simulink library "aerolibtransform"  (Simulink 5.0)
libraries: simulink x5, aerolibtransform x2, aerolibutil x2, simulink3 x1
settings Model: Creator=sgage  LastModifiedBy=sgage  ExtModeAutoUpdateStatusClock=off  TargetHWChar=2  TargetHWWordLengths=8,16,32,32
settings Model: ForwardingTableString=|
  | ||__slOldName__||aerolibtransform/Direction Cosine Matrix to
  | Euler Angles||__slNewName__||aerolibtransform2/Direction Cosine Matrix to
  | Euler Angles||__slOldName__||aerolibtransform/Euler Angles to
  | Direction Cosine Matrix||__slNewName__||aerolibtransform2/Euler Angles to
  | Direction Cosine Matrix||__slOldName__||aerolibtransform/Direction Cosine Matrix
  | to Quaternions||__slNewName__||aerolibtransform2/Direction Cosine Matrix
  | to Quaternions||__slOldName__||aerolibtransform/Quaternions to
  | Direction Cosine Matrix||__slNewName__||aerolibtransform2/Quaternions to
  | Direction Cosine Matrix||__slOldName__||aerolibtransform/Euler Angles to Quaternions||__slNewName__||aerolibtransform2/Euler Angles to Quaternions||__slOldName__||aerolibtransform/Quaternions to Euler Angles||__slNewName__||aerolibtransform2/Quaternions to Euler Angles||__slOldName__||aerolibtransform/3x3 Cross Product||__slNewName__||aerolibutil/3x3 Cross Product

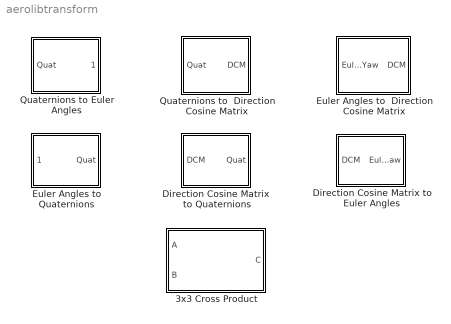
== system aerolibtransform ==
  3x3 Cross Product : Subsystem
      mask Type: CrossProduct
      mask Description: Calculate the cross product of two 3-by-1 vectors.
      mask Help: web(asbhelp('3x3crossproduct'));
      mask Display: disp('Cross Product \n C = AxB')
  Direction Cosine Matrix  to Quaternions : Subsystem
      mask Type: DCM2Quaternion
      mask Description: Determine the 4x1 quaternion orientation vector from a 3-by-3 direction cosine matrix (DCM). The input DCM transforms vectors from inertial axes to body axes.
      mask Help: web(asbhelp('directioncosinematrixtoquaternions'));
      mask Display: disp('DCM2Quat')
  Direction Cosine Matrix to Euler Angles : Subsystem
      mask Type: DCM2Euler
      mask Description: Determine an euler orientation (roll, pitch, yaw) from the 3-by-3 direction cosine matrix (DCM). The input DCM transforms vectors from inertial axes to body axes.
      mask Help: web(asbhelp('directioncosinematrixtoeulerangles'));
      mask Display: disp('DCM2Eul')
  Euler Angles to  Direction Cosine Matrix : Subsystem
      mask Type: Euler2DCM
      mask Description: Determine the 3-by-3 direction cosine matrix (DCM) from an Euler orientation (roll, pitch, yaw). The output DCM transforms vectors from inertial axes to body axes.
      mask Help: web(asbhelp('euleranglestodirectioncosinematrix'));
      mask Display: disp('Eul2DCM')
  Euler Angles to Quaternions : Subsystem
      mask Type: Euler2Quaternion
      mask Description: Calculate quaternion (q0,q1,q2,q3) from Euler angles (roll, pitch, yaw)
      mask Help: web(asbhelp('euleranglestoquaternions'));
      mask Display: disp('Eul2Quat')
  Quaternions to  Direction Cosine Matrix : Subsystem
      mask Type: Quaternion2DCM
      mask Description: Determine the 3-by-3 direction cosine matrix (DCM) from a 4-by-1 quaternion orientation vector. The output DCM transforms vectors from inertial axes to body axes.
      mask Help: web(asbhelp('quaternionstodirectioncosinematrix'));
      mask Display: disp('Quat2DCM')
  Quaternions to Euler Angles : Subsystem
      mask Type: Quaternion2Euler
      mask Description: Calculate Euler angles (roll, pitch, yaw) from quaternion (q0,q1,q2,q3)
      mask Help: web(asbhelp('quaternionstoeulerangles'));
      mask Display: disp('Quat2Eul')

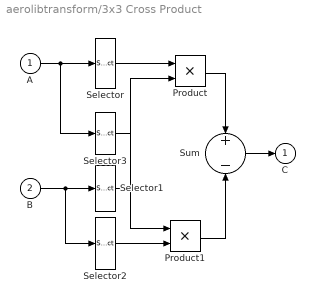
== system aerolibtransform/3x3 Cross Product ==
  A : Inport
  B : Inport  Port=2
  Product : Product  SaturateOnIntegerOverflow=on  InputSameDT=on
  Product1 : Product  SaturateOnIntegerOverflow=on  InputSameDT=on
  Selector : Selector  Elements=[2 3 1]  InputPortWidth=3
  Selector1 : Selector  Elements=[3 1 2]  InputPortWidth=3
  Selector2 : Selector  Elements=[2 3 1]  InputPortWidth=3
  Selector3 : Selector  Elements=[3 1 2]  InputPortWidth=3
  Sum : Sum  Inputs=+|-  SaturateOnIntegerOverflow=on  InputSameDT=on
  C : Outport  InitialOutput=0
  wires:
  Selector3/1 -> Product1/1
  Selector2/1 -> Product1/2
  Product1/1 -> Sum/2
  Selector1/1 -> Product/2
  Product/1 -> Sum/1
  A/1 -> Selector3/1, Selector/1
  Selector/1 -> Product/1
  B/1 -> Selector2/1, Selector1/1
  Sum/1 -> C/1

== system aerolibtransform/Direction Cosine Matrix  to Quaternions ==
  DCM : Inport
  If : If
  Merge : Merge
  Negative Trace : Subsystem  TreatAsAtomicUnit=on
  Positive Trace : Subsystem  TreatAsAtomicUnit=on
  "Reshape 3x3 -> 9x1" : simulink/Math Operations/Reshape  OutputDimensionality=Customize  OutputDimensions=[9,1]
  trace(DCM) : Fcn  Expr=u(1)+u(5)+u(9)
  Quat : Outport
  wires:
  If/2 -> Negative Trace/Action
  If/1 -> Positive Trace/Action
  Negative Trace/1(qw qx qy qz) -> Merge/2
  DCM/1 -> "Reshape 3x3 -> 9x1"/1
  "Reshape 3x3 -> 9x1"/1 -> trace(DCM)/1, Positive Trace/2(DCM), Negative Trace/1(DCM)
  trace(DCM)/1 -> If/1, Positive Trace/1(trace(DCM))
  Positive Trace/1(qw qx qy qz) -> Merge/1
  Merge/1 -> Quat/1

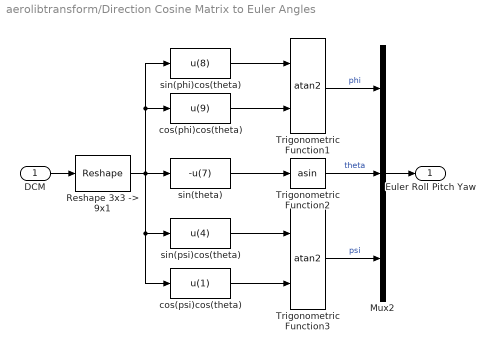
== system aerolibtransform/Direction Cosine Matrix to Euler Angles ==
  DCM : Inport
  Mux2 : Mux  Inputs=3
  "Reshape 3x3 -> 9x1" : simulink/Math Operations/Reshape  OutputDimensionality=Customize  OutputDimensions=[9, 1]
  Trigonometric Function1 : Trigonometry  Operator=atan2
  Trigonometric Function2 : Trigonometry  Operator=asin
  Trigonometric Function3 : Trigonometry  Operator=atan2
  cos(phi)cos(theta) : Fcn  Expr=u(9)
  cos(psi)cos(theta) : Fcn  Expr=u(1)
  sin(phi)cos(theta) : Fcn  Expr=u(8)
  sin(psi)cos(theta) : Fcn  Expr=u(4)
  sin(theta) : Fcn  Expr=-u(7)
  Euler Roll Pitch Yaw : Outport  InitialOutput=0
  wires:
  Mux2/1 -> Euler Roll Pitch Yaw/1
  Trigonometric Function3/1 -> Mux2/3  "psi"
  Trigonometric Function2/1 -> Mux2/2  "theta"
  Trigonometric Function1/1 -> Mux2/1  "phi"
  cos(psi)cos(theta)/1 -> Trigonometric Function3/2
  sin(psi)cos(theta)/1 -> Trigonometric Function3/1
  cos(phi)cos(theta)/1 -> Trigonometric Function1/2
  sin(phi)cos(theta)/1 -> Trigonometric Function1/1
  sin(theta)/1 -> Trigonometric Function2/1
  "Reshape 3x3 -> 9x1"/1 -> cos(psi)cos(theta)/1, sin(psi)cos(theta)/1, cos(phi)cos(theta)/1, sin(phi)cos(theta)/1, sin(theta)/1
  DCM/1 -> "Reshape 3x3 -> 9x1"/1

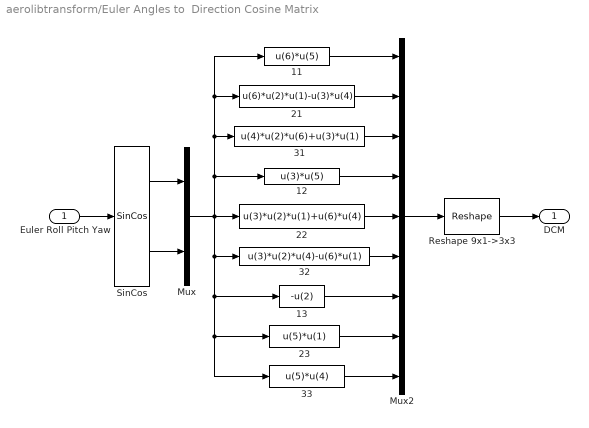
== system aerolibtransform/Euler Angles to  Direction Cosine Matrix ==
  Euler Roll Pitch Yaw : Inport
  11 : Fcn  Expr=u(6)*u(5)
  12 : Fcn  Expr=u(3)*u(5)
  13 : Fcn  Expr=-u(2)
  21 : Fcn  Expr=u(6)*u(2)*u(1)-u(3)*u(4)
  22 : Fcn  Expr=u(3)*u(2)*u(1)+u(6)*u(4)
  23 : Fcn  Expr=u(5)*u(1)
  31 : Fcn  Expr=u(4)*u(2)*u(6)+u(3)*u(1)
  32 : Fcn  Expr=u(3)*u(2)*u(4)-u(6)*u(1)
  33 : Fcn  Expr=u(5)*u(4)
  Mux : Mux  Inputs=2
  Mux2 : Mux  Inputs=9
  Reshape 9x1->3x3 : simulink/Math Operations/Reshape  OutputDimensionality=Customize  OutputDimensions=[3,3]
  SinCos : aerolibutil/SinCos
  DCM : Outport  InitialOutput=0
  wires:
  Mux/1 -> 33/1, 23/1, 13/1, 32/1, 12/1, 31/1, 21/1, 11/1, 22/1
  SinCos/2 -> Mux/2
  SinCos/1 -> Mux/1
  Reshape 9x1->3x3/1 -> DCM/1
  Mux2/1 -> Reshape 9x1->3x3/1
  11/1 -> Mux2/1
  21/1 -> Mux2/2
  31/1 -> Mux2/3
  12/1 -> Mux2/4
  22/1 -> Mux2/5
  32/1 -> Mux2/6
  13/1 -> Mux2/7
  23/1 -> Mux2/8
  33/1 -> Mux2/9
  Euler Roll Pitch Yaw/1 -> SinCos/1

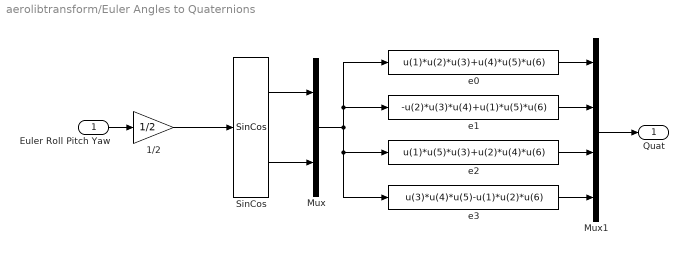
== system aerolibtransform/Euler Angles to Quaternions ==
  Euler Roll Pitch Yaw : Inport
  1/2 : Gain  Gain=1/2  SaturateOnIntegerOverflow=on
  Mux : Mux  Inputs=2
  Mux1 : Mux
  SinCos : aerolibutil/SinCos
  e0 : Fcn  Expr=u(1)*u(2)*u(3)+u(4)*u(5)*u(6)
  e1 : Fcn  Expr=-u(2)*u(3)*u(4)+u(1)*u(5)*u(6)
  e2 : Fcn  Expr=u(1)*u(5)*u(3)+u(2)*u(4)*u(6)
  e3 : Fcn  Expr=u(3)*u(4)*u(5)-u(1)*u(2)*u(6)
  Quat : Outport  InitialOutput=0
  wires:
  Mux1/1 -> Quat/1
  e3/1 -> Mux1/4
  e2/1 -> Mux1/3
  e1/1 -> Mux1/2
  e0/1 -> Mux1/1
  Mux/1 -> e0/1, e1/1, e3/1, e2/1
  SinCos/2 -> Mux/2
  SinCos/1 -> Mux/1
  Euler Roll Pitch Yaw/1 -> 1/2/1
  1/2/1 -> SinCos/1

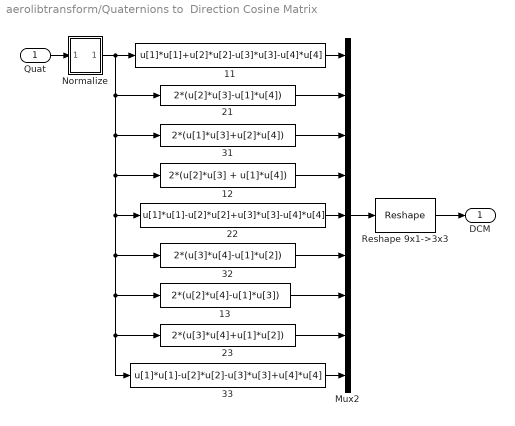
== system aerolibtransform/Quaternions to  Direction Cosine Matrix ==
  Quat : Inport
  11 : Fcn  Expr=u[1]*u[1]+u[2]*u[2]-u[3]*u[3]-u[4]*u[4]
  12 : Fcn  Expr=2*(u[2]*u[3] + u[1]*u[4])
  13 : Fcn  Expr=2*(u[2]*u[4]-u[1]*u[3])
  21 : Fcn  Expr=2*(u[2]*u[3]-u[1]*u[4])
  22 : Fcn  Expr=u[1]*u[1]-u[2]*u[2]+u[3]*u[3]-u[4]*u[4]
  23 : Fcn  Expr=2*(u[3]*u[4]+u[1]*u[2])
  31 : Fcn  Expr=2*(u[1]*u[3]+u[2]*u[4])
  32 : Fcn  Expr=2*(u[3]*u[4]-u[1]*u[2])
  33 : Fcn  Expr=u[1]*u[1]-u[2]*u[2]-u[3]*u[3]+u[4]*u[4]
  Mux2 : Mux  Inputs=9
  Normalize : Subsystem
  Reshape 9x1->3x3 : simulink/Math Operations/Reshape  OutputDimensionality=Customize  OutputDimensions=[3,3]
  DCM : Outport  InitialOutput=0
  wires:
  Mux2/1 -> Reshape 9x1->3x3/1
  Reshape 9x1->3x3/1 -> DCM/1
  11/1 -> Mux2/1
  21/1 -> Mux2/2
  31/1 -> Mux2/3
  12/1 -> Mux2/4
  22/1 -> Mux2/5
  32/1 -> Mux2/6
  13/1 -> Mux2/7
  23/1 -> Mux2/8
  33/1 -> Mux2/9
  Quat/1 -> Normalize/1(In1)
  Normalize/1(Out1) -> 11/1, 21/1, 31/1, 12/1, 22/1, 32/1, 13/1, 33/1, 23/1

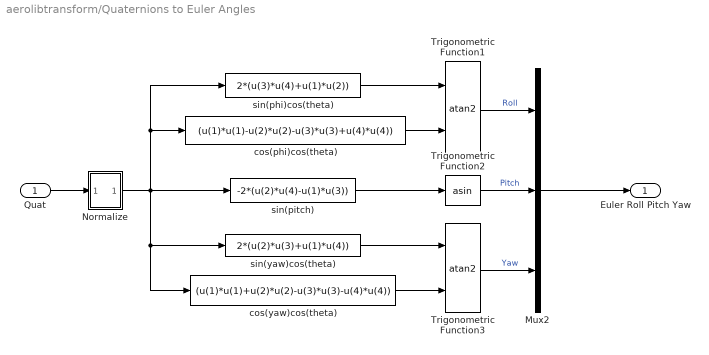
== system aerolibtransform/Quaternions to Euler Angles ==
  Quat : Inport
  Mux2 : Mux  Inputs=3
  Normalize : Subsystem
  Trigonometric Function1 : Trigonometry  Operator=atan2
  Trigonometric Function2 : Trigonometry  Operator=asin
  Trigonometric Function3 : Trigonometry  Operator=atan2
  cos(phi)cos(theta) : Fcn  Expr=(u(1)*u(1)-u(2)*u(2)-u(3)*u(3)+u(4)*u(4))
  cos(yaw)cos(theta) : Fcn  Expr=(u(1)*u(1)+u(2)*u(2)-u(3)*u(3)-u(4)*u(4))
  sin(phi)cos(theta) : Fcn  Expr=2*(u(3)*u(4)+u(1)*u(2))
  sin(pitch) : Fcn  Expr=-2*(u(2)*u(4)-u(1)*u(3))
  sin(yaw)cos(theta) : Fcn  Expr=2*(u(2)*u(3)+u(1)*u(4))
  Euler Roll Pitch Yaw : Outport  InitialOutput=0
  wires:
  Quat/1 -> Normalize/1(In1)
  Normalize/1(Out1) -> cos(phi)cos(theta)/1, sin(phi)cos(theta)/1, sin(pitch)/1, cos(yaw)cos(theta)/1, sin(yaw)cos(theta)/1
  Trigonometric Function2/1 -> Mux2/2  "Pitch"
  Mux2/1 -> Euler Roll Pitch Yaw/1
  sin(pitch)/1 -> Trigonometric Function2/1
  Trigonometric Function1/1 -> Mux2/1  "Roll"
  sin(phi)cos(theta)/1 -> Trigonometric Function1/1
  cos(phi)cos(theta)/1 -> Trigonometric Function1/2
  Trigonometric Function3/1 -> Mux2/3  "Yaw"
  sin(yaw)cos(theta)/1 -> Trigonometric Function3/1
  cos(yaw)cos(theta)/1 -> Trigonometric Function3/2

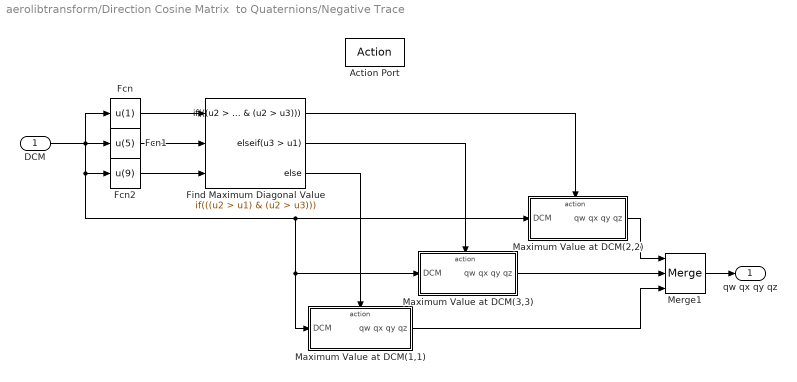
== system aerolibtransform/Direction Cosine Matrix  to Quaternions/Negative Trace ==
  DCM : Inport
  Action Port : ActionPort
  Fcn : Fcn  Expr=u(1)
  Fcn1 : Fcn  Expr=u(5)
  Fcn2 : Fcn  Expr=u(9)
  Find Maximum Diagonal Value : If  NumInputs=3  IfExpression=((u2 > u1) & (u2 > u3))  ElseIfExpressions=u3 > u1
  Maximum Value at DCM(1,1) : Subsystem  TreatAsAtomicUnit=on
  Maximum Value at DCM(2,2) : Subsystem  TreatAsAtomicUnit=on
  Maximum Value at DCM(3,3) : Subsystem  TreatAsAtomicUnit=on
  Merge1 : Merge  Inputs=3
  qw qx qy qz : Outport
  wires:
  Fcn2/1 -> Find Maximum Diagonal Value/3
  Fcn1/1 -> Find Maximum Diagonal Value/2
  Fcn/1 -> Find Maximum Diagonal Value/1
  DCM/1 -> Fcn2/1, Maximum Value at DCM(2,2)/1(DCM), Maximum Value at DCM(3,3)/1(DCM), Maximum Value at DCM(1,1)/1(DCM), Fcn1/1, Fcn/1
  Find Maximum Diagonal Value/3 -> Maximum Value at DCM(1,1)/Action
  Maximum Value at DCM(2,2)/1(qw qx qy qz) -> Merge1/1
  Maximum Value at DCM(3,3)/1(qw qx qy qz) -> Merge1/2
  Maximum Value at DCM(1,1)/1(qw qx qy qz) -> Merge1/3
  Merge1/1 -> qw qx qy qz/1
  Find Maximum Diagonal Value/1 -> Maximum Value at DCM(2,2)/Action
  Find Maximum Diagonal Value/2 -> Maximum Value at DCM(3,3)/Action

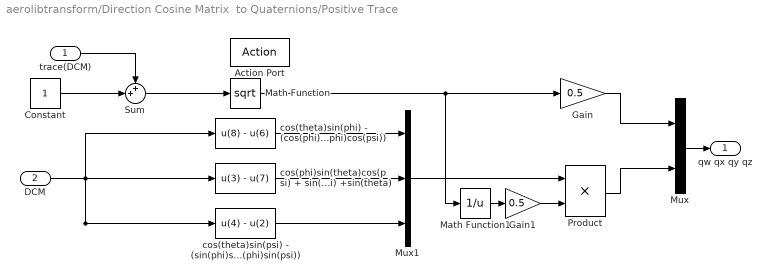
== system aerolibtransform/Direction Cosine Matrix  to Quaternions/Positive Trace ==
  trace(DCM) : Inport
  DCM : Inport  Port=2
  Action Port : ActionPort
  Constant : Constant  ShowAdditionalParam=on
  Gain : Gain  Gain=0.5  ShowAdditionalParam=on  SaturateOnIntegerOverflow=on
  Gain1 : Gain  Gain=0.5  ShowAdditionalParam=on  SaturateOnIntegerOverflow=on
  Math Function : Math  Operator=sqrt
  Math Function1 : Math  Operator=reciprocal
  Mux : Mux  Inputs=2
  Mux1 : Mux  Inputs=3
  Product : Product  ShowAdditionalParam=on  SaturateOnIntegerOverflow=on  InputSameDT=on
  Sum : Sum  Inputs=++|  ShowAdditionalParam=on  SaturateOnIntegerOverflow=on  InputSameDT=on
  cos(phi)sin(theta)cos(psi) + sin(phi)sin(psi) +sin(theta) : Fcn  Expr=u(3) - u(7)
  cos(theta)sin(phi) - (cos(phi)sin(theta)sin(psi) - sin(phi)cos(psi)) : Fcn  Expr=u(8) - u(6)
  cos(theta)sin(psi) - (sin(phi)sin(theta)cos(psi) - cos(phi)sin(psi)) : Fcn  Expr=u(4) - u(2)
  qw qx qy qz : Outport
  wires:
  Math Function/1 -> Gain/1, Math Function1/1
  Sum/1 -> Math Function/1
  Mux/1 -> qw qx qy qz/1
  cos(theta)sin(psi) - (sin(phi)sin(theta)cos(psi) - cos(phi)sin(psi))/1 -> Mux1/3
  cos(phi)sin(theta)cos(psi) + sin(phi)sin(psi) +sin(theta)/1 -> Mux1/2
  cos(theta)sin(phi) - (cos(phi)sin(theta)sin(psi) - sin(phi)cos(psi))/1 -> Mux1/1
  DCM/1 -> cos(theta)sin(phi) - (cos(phi)sin(theta)sin(psi) - sin(phi)cos(psi))/1, cos(phi)sin(theta)cos(psi) + sin(phi)sin(psi) +sin(theta)/1, cos(theta)sin(psi) - (sin(phi)sin(theta)cos(psi) - cos(phi)sin(psi))/1
  Math Function1/1 -> Gain1/1
  Gain/1 -> Mux/1
  Mux1/1 -> Product/1
  Gain1/1 -> Product/2
  Constant/1 -> Sum/2
  trace(DCM)/1 -> Sum/1
  Product/1 -> Mux/2

== system aerolibtransform/Quaternions to  Direction Cosine Matrix/Normalize ==
  In1 : Inport
  Dot Product : simulink/Math Operations/Dot Product
  Math Function : Math  Operator=sqrt
  Normalize Quaternion Magnitude : Product  Inputs=*/  SaturateOnIntegerOverflow=on  InputSameDT=on
  Out1 : Outport
  wires:
  In1/1 -> Normalize Quaternion Magnitude/1, Dot Product/2, Dot Product/1
  Dot Product/1 -> Math Function/1
  Math Function/1 -> Normalize Quaternion Magnitude/2
  Normalize Quaternion Magnitude/1 -> Out1/1

== system aerolibtransform/Quaternions to Euler Angles/Normalize ==
  In1 : Inport
  Dot Product : simulink3/Math/Dot Product
  Math Function : Math  Operator=sqrt
  Normalize Quaternion Magnitude : Product  Inputs=*/  SaturateOnIntegerOverflow=on  InputSameDT=on
  Out1 : Outport
  wires:
  Normalize Quaternion Magnitude/1 -> Out1/1
  Math Function/1 -> Normalize Quaternion Magnitude/2
  Dot Product/1 -> Math Function/1
  In1/1 -> Dot Product/1, Dot Product/2, Normalize Quaternion Magnitude/1

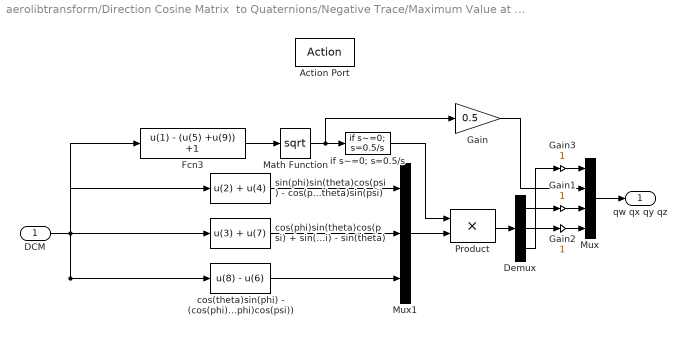
== system aerolibtransform/Direction Cosine Matrix  to Quaternions/Negative Trace/Maximum Value at DCM(1,1) ==
  DCM : Inport
  Action Port : ActionPort
  " sin(phi)sin(theta)cos(psi) - cos(phi)sin(psi) + cos(theta)sin(psi)" : Fcn  Expr=u(2) + u(4)
  Demux : Demux  Outputs=3
  Fcn3 : Fcn  Expr=u(1) - (u(5) +u(9)) +1
  Gain : Gain  Gain=0.5  SaturateOnIntegerOverflow=on
  Gain1 : Gain  SaturateOnIntegerOverflow=on
  Gain2 : Gain  SaturateOnIntegerOverflow=on
  Gain3 : Gain  SaturateOnIntegerOverflow=on
  Math Function : Math  Operator=sqrt
  Mux : Mux
  Mux1 : Mux  Inputs=3
  Product : Product  SaturateOnIntegerOverflow=on  InputSameDT=on
  cos(phi)sin(theta)cos(psi) + sin(phi)sin(psi) - sin(theta) : Fcn  Expr=u(3) + u(7)
  cos(theta)sin(phi) - (cos(phi)sin(theta)sin(psi) - sin(phi)cos(psi)) : Fcn  Expr=u(8) - u(6)
  if s~=0; s=0.5/s : aerolibtransform/Direction Cosine Matrix  to Quaternions/Negative Trace/Maximum Value at DCM(2,2)/if s~=0; s=0.5//s  SimViewingDevice=off  DataTypeOverride=UseLocalSettings  MinMaxOverflowLogging=UseLocalSettings
      settings: Permissions=ReadWrite  RTWFcnNameOpts=Auto  RTWFileNameOpts=Auto
  qw qx qy qz : Outport
  wires:
  DCM/1 -> " sin(phi)sin(theta)cos(psi) - cos(phi)sin(psi) + cos(theta)sin(psi)"/1, cos(phi)sin(theta)cos(psi) + sin(phi)sin(psi) - sin(theta)/1, cos(theta)sin(phi) - (cos(phi)sin(theta)sin(psi) - sin(phi)cos(psi))/1, Fcn3/1
  " sin(phi)sin(theta)cos(psi) - cos(phi)sin(psi) + cos(theta)sin(psi)"/1 -> Mux1/1
  cos(phi)sin(theta)cos(psi) + sin(phi)sin(psi) - sin(theta)/1 -> Mux1/2
  cos(theta)sin(phi) - (cos(phi)sin(theta)sin(psi) - sin(phi)cos(psi))/1 -> Mux1/3
  Mux/1 -> qw qx qy qz/1
  Fcn3/1 -> Math Function/1
  Math Function/1 -> if s~=0; s=0.5/s/1, Gain/1
  Mux1/1 -> Product/2
  Demux/1 -> Gain1/1
  Demux/3 -> Gain3/1
  Demux/2 -> Gain2/1
  Gain1/1 -> Mux/3
  Gain2/1 -> Mux/4
  Gain3/1 -> Mux/1
  Product/1 -> Demux/1
  Gain/1 -> Mux/2
  if s~=0; s=0.5/s/1 -> Product/1

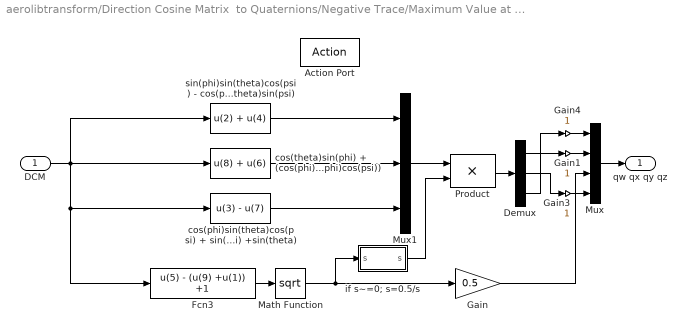
== system aerolibtransform/Direction Cosine Matrix  to Quaternions/Negative Trace/Maximum Value at DCM(2,2) ==
  DCM : Inport
  Action Port : ActionPort
  " sin(phi)sin(theta)cos(psi) - cos(phi)sin(psi) + cos(theta)sin(psi)" : Fcn  Expr=u(2) + u(4)
  Demux : Demux  Outputs=3
  Fcn3 : Fcn  Expr=u(5) - (u(9) +u(1)) +1
  Gain : Gain  Gain=0.5  SaturateOnIntegerOverflow=on
  Gain1 : Gain  SaturateOnIntegerOverflow=on
  Gain3 : Gain  SaturateOnIntegerOverflow=on
  Gain4 : Gain  SaturateOnIntegerOverflow=on
  Math Function : Math  Operator=sqrt
  Mux : Mux
  Mux1 : Mux  Inputs=3
  Product : Product  SaturateOnIntegerOverflow=on  InputSameDT=on
  cos(phi)sin(theta)cos(psi) + sin(phi)sin(psi) +sin(theta) : Fcn  Expr=u(3) - u(7)
  cos(theta)sin(phi) + (cos(phi)sin(theta)sin(psi) - sin(phi)cos(psi)) : Fcn  Expr=u(8) + u(6)
  if s~=0; s=0.5/s : Subsystem
  qw qx qy qz : Outport
  wires:
  Mux1/1 -> Product/1
  DCM/1 -> Fcn3/1, cos(phi)sin(theta)cos(psi) + sin(phi)sin(psi) +sin(theta)/1, " sin(phi)sin(theta)cos(psi) - cos(phi)sin(psi) + cos(theta)sin(psi)"/1, cos(theta)sin(phi) + (cos(phi)sin(theta)sin(psi) - sin(phi)cos(psi))/1
  " sin(phi)sin(theta)cos(psi) - cos(phi)sin(psi) + cos(theta)sin(psi)"/1 -> Mux1/1
  cos(theta)sin(phi) + (cos(phi)sin(theta)sin(psi) - sin(phi)cos(psi))/1 -> Mux1/2
  cos(phi)sin(theta)cos(psi) + sin(phi)sin(psi) +sin(theta)/1 -> Mux1/3
  Mux/1 -> qw qx qy qz/1
  Fcn3/1 -> Math Function/1
  Gain/1 -> Mux/3
  Product/1 -> Demux/1
  Demux/1 -> Gain1/1
  Demux/2 -> Gain3/1
  Demux/3 -> Gain4/1
  Gain1/1 -> Mux/2
  Gain3/1 -> Mux/4
  Gain4/1 -> Mux/1
  if s~=0; s=0.5/s/1("s ") -> Product/2
  Math Function/1 -> if s~=0; s=0.5/s/1(s), Gain/1

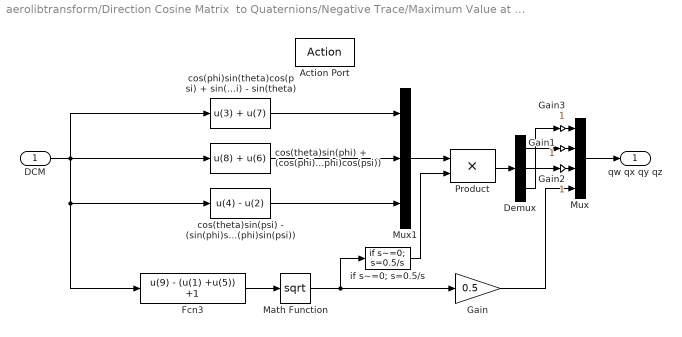
== system aerolibtransform/Direction Cosine Matrix  to Quaternions/Negative Trace/Maximum Value at DCM(3,3) ==
  DCM : Inport
  Action Port : ActionPort
  Demux : Demux  Outputs=3
  Fcn3 : Fcn  Expr=u(9) - (u(1) +u(5)) +1
  Gain : Gain  Gain=0.5  SaturateOnIntegerOverflow=on
  Gain1 : Gain  SaturateOnIntegerOverflow=on
  Gain2 : Gain  SaturateOnIntegerOverflow=on
  Gain3 : Gain  SaturateOnIntegerOverflow=on
  Math Function : Math  Operator=sqrt
  Mux : Mux
  Mux1 : Mux  Inputs=3
  Product : Product  SaturateOnIntegerOverflow=on  InputSameDT=on
  cos(phi)sin(theta)cos(psi) + sin(phi)sin(psi) - sin(theta) : Fcn  Expr=u(3) + u(7)
  cos(theta)sin(phi) + (cos(phi)sin(theta)sin(psi) - sin(phi)cos(psi)) : Fcn  Expr=u(8) + u(6)
  cos(theta)sin(psi) - (sin(phi)sin(theta)cos(psi) - cos(phi)sin(psi)) : Fcn  Expr=u(4) - u(2)
  if s~=0; s=0.5/s : aerolibtransform/Direction Cosine Matrix  to Quaternions/Negative Trace/Maximum Value at DCM(2,2)/if s~=0; s=0.5//s  SimViewingDevice=off  DataTypeOverride=UseLocalSettings  MinMaxOverflowLogging=UseLocalSettings
      settings: Permissions=ReadWrite  RTWFcnNameOpts=Auto  RTWFileNameOpts=Auto
  qw qx qy qz : Outport
  wires:
  Mux1/1 -> Product/1
  DCM/1 -> cos(phi)sin(theta)cos(psi) + sin(phi)sin(psi) - sin(theta)/1, cos(theta)sin(phi) + (cos(phi)sin(theta)sin(psi) - sin(phi)cos(psi))/1, cos(theta)sin(psi) - (sin(phi)sin(theta)cos(psi) - cos(phi)sin(psi))/1, Fcn3/1
  cos(phi)sin(theta)cos(psi) + sin(phi)sin(psi) - sin(theta)/1 -> Mux1/1
  cos(theta)sin(phi) + (cos(phi)sin(theta)sin(psi) - sin(phi)cos(psi))/1 -> Mux1/2
  cos(theta)sin(psi) - (sin(phi)sin(theta)cos(psi) - cos(phi)sin(psi))/1 -> Mux1/3
  Mux/1 -> qw qx qy qz/1
  Fcn3/1 -> Math Function/1
  Math Function/1 -> if s~=0; s=0.5/s/1, Gain/1
  Product/1 -> Demux/1
  Demux/1 -> Gain1/1
  Demux/3 -> Gain3/1
  Demux/2 -> Gain2/1
  Gain/1 -> Mux/4
  Gain1/1 -> Mux/2
  Gain2/1 -> Mux/3
  Gain3/1 -> Mux/1
  if s~=0; s=0.5/s/1 -> Product/2

== system aerolibtransform/Direction Cosine Matrix  to Quaternions/Negative Trace/Maximum Value at DCM(2,2)/if s~=0; s=0.5/s ==
  s : Inport
  Constant : Constant  Value=0  ShowAdditionalParam=on
  Gain2 : Gain  Gain=0.5  SaturateOnIntegerOverflow=on
  Math Function1 : Math  Operator=reciprocal
  Relational Operator : RelationalOperator  Operator=~=  InputSameDT=on
  Switch : Switch  Threshold=0.5  SaturateOnIntegerOverflow=on  InputSameDT=on
  "s " : Outport
  wires:
  Math Function1/1 -> Gain2/1
  Gain2/1 -> Switch/1
  Relational Operator/1 -> Switch/2
  Constant/1 -> Relational Operator/2
  s/1 -> Math Function1/1, Relational Operator/1, Switch/3
  Switch/1 -> "s "/1
